simulink model "control_4_channels"  (R2024a)
settings: Solver=FixedStepAuto  StartTime=0.0  StopTime=10.0  FixedStep=0.002  RelTol=1e-3  EnableMultiTasking=on
settings Model: ExtModeTrigDuration=2  Creator=Jesper  LastModifiedBy=20215368
settings SolverCC: PositivePriorityOrder=on
settings OptimizationCC: EnhancedBackFolding=on  PassReuseOutputArgsAs=Individual arguments  ZeroExternalMemoryAtStartup=off  ZeroInternalMemoryAtStartup=off  MaxStackSize=64  OptimizeBlockOrder=speed  DifferentSizesBufferReuse=on  OptimizationCustomize=off  EfficientTunableParamExpr=on
settings DebuggingCC: ParameterTunabilityLossMsg=error
settings HardwareCC: ProdBitPerPointer=32  ProdBitPerSizeT=32  ProdBitPerPtrDiffT=32  ProdLargestAtomicInteger=Long  ProdLargestAtomicFloat=Double  ProdWordSize=32  ProdLongLongMode=on  ProdHWDeviceType=ARM Compatible->ARM Cortex  UseEmbeddedCoderFeatures=off
settings RTWCC: Description=Embedded Coder  SystemTargetFile=ert.tlc  HardwareBoard=Raspberry Pi  TLCOptions="-aInlineSetEventsForThisBaseRateFcn=TLC_FALSE -aSuppressMultiTaskScheduler=TLC_FALSE  -aRateBasedStepFcn=0"  TemplateMakefile=ert_default_tmf  Toolchain=GNU GCC Embedded Linux  BuildConfiguration=Faster Runs
settings CodeAppCC: ForceParamTrailComments=on  IgnoreCustomStorageClasses=off  OperatorAnnotations=on  SimulinkDataObjDesc=on  SFDataObjDesc=on  InsertBlockDesc=on
settings ERTTargetCC: SupportNonInlinedSFcns=on  SupportVariableSizeSignals=on  ExtModeTransport=2  ExtModeStaticAlloc=on  ExtModeMexFile=ext_xcp  ExtModeIntrfLevel=Level2 - Open

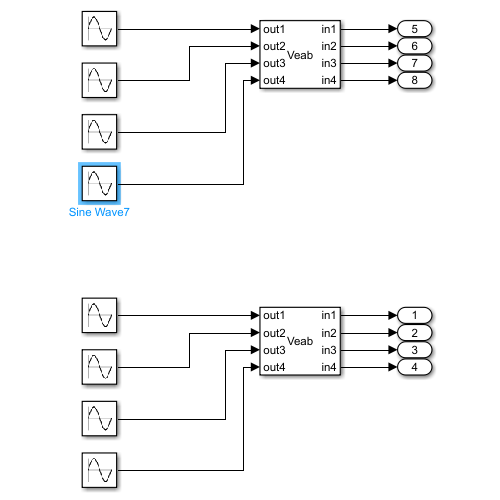
[thumbnail: Simulink's stored preview of the top-level diagram]
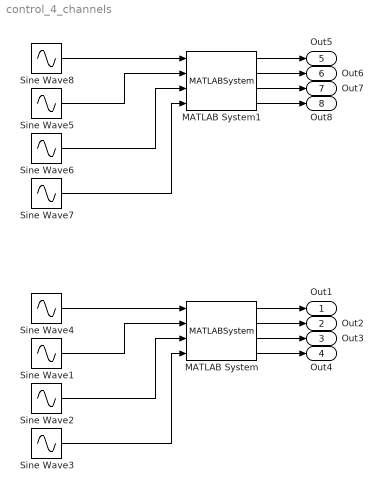
== system control_4_channels ==
  MATLAB System : MATLABSystem  System=Veab  i2cbus=1  resolution=0.002578125
      mask Type: Veab
      mask Display:
      | disp('Veab');
      | port_label('input',1,'out1');
      | port_label('input',2,'out2');
      | port_label('input',3,'out3');
      | port_label('input',4,'out4');
      | port_label('output',1,'in1');
      | port_label('output',2,'in2');
      | port_label('output',3,'in3');
      | port_label('output',4,'in4');
  MATLAB System1 : MATLABSystem  System=Veab  i2cbus=3  resolution=0.002578125
      mask Type: Veab
      mask Display:
      | disp('Veab');
      | port_label('input',1,'out1');
      | port_label('input',2,'out2');
      | port_label('input',3,'out3');
      | port_label('input',4,'out4');
      | port_label('output',1,'in1');
      | port_label('output',2,'in2');
      | port_label('output',3,'in3');
      | port_label('output',4,'in4');
  Sine Wave1 : Sin  Amplitude=5  Bias=5  Frequency=2  SampleTime=0
  Sine Wave2 : Sin  Amplitude=5  Bias=5  Frequency=4  SampleTime=0
  Sine Wave3 : Sin  Amplitude=5  Bias=5  Frequency=8  SampleTime=0
  Sine Wave4 : Sin  Amplitude=5  Bias=5  SampleTime=0
  Sine Wave5 : Sin  Amplitude=3  Bias=5  Frequency=2  SampleTime=0
  Sine Wave6 : Sin  Amplitude=3  Bias=5  Frequency=4  SampleTime=0
  Sine Wave7 : Sin  Amplitude=3  Bias=5  Frequency=8  SampleTime=0
  Sine Wave8 : Sin  Amplitude=3  Bias=5  SampleTime=0
  Out1 : Outport
  Out2 : Outport  Port=2
  Out3 : Outport  Port=3
  Out4 : Outport  Port=4
  Out5 : Outport  Port=5
  Out6 : Outport  Port=6
  Out7 : Outport  Port=7
  Out8 : Outport  Port=8
  wires:
  Sine Wave1/1 -> MATLAB System/2
  Sine Wave2/1 -> MATLAB System/3
  Sine Wave3/1 -> MATLAB System/4
  MATLAB System/1 -> Out1/1
  MATLAB System/2 -> Out2/1
  MATLAB System/3 -> Out3/1
  MATLAB System/4 -> Out4/1
  Sine Wave4/1 -> MATLAB System/1
  MATLAB System1/2 -> Out6/1
  Sine Wave8/1 -> MATLAB System1/1
  Sine Wave6/1 -> MATLAB System1/3
  Sine Wave5/1 -> MATLAB System1/2
  MATLAB System1/3 -> Out7/1
  Sine Wave7/1 -> MATLAB System1/4
  MATLAB System1/1 -> Out5/1
  MATLAB System1/4 -> Out8/1
